simulink model "Copy_of_Facies"  (R2023a)
settings: Solver=VariableStepAuto  StartTime=0.0  StopTime=6  RelTol=1e-3
(part 1 of 2)
settings Model: Creator=Stefano  LastModifiedBy=stefanopanzieri
settings SolverCC: AlgebraicLoopSolver=TrustRegion
settings DebuggingCC: UnconnectedInputMsg=warning  UnconnectedOutputMsg=warning  UnconnectedLineMsg=warning
settings ModelReferenceCC: EnableRefExpFcnMdlSchedulingChecks=on
settings SFSimCC: CustomCodeUndefinedFunction=UseInterfaceOnly
settings RTWCC: DLArmComputeVersion=19.05

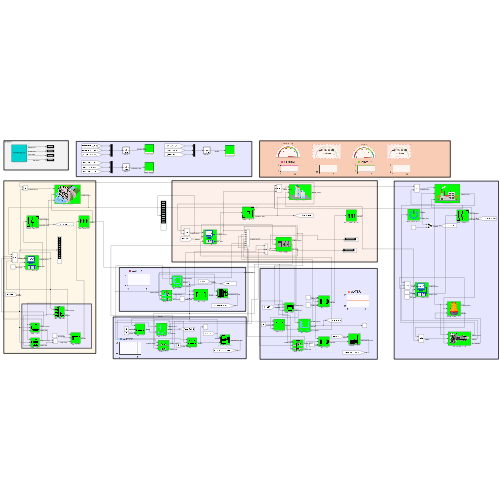
[thumbnail: Simulink's stored preview of the top-level diagram]
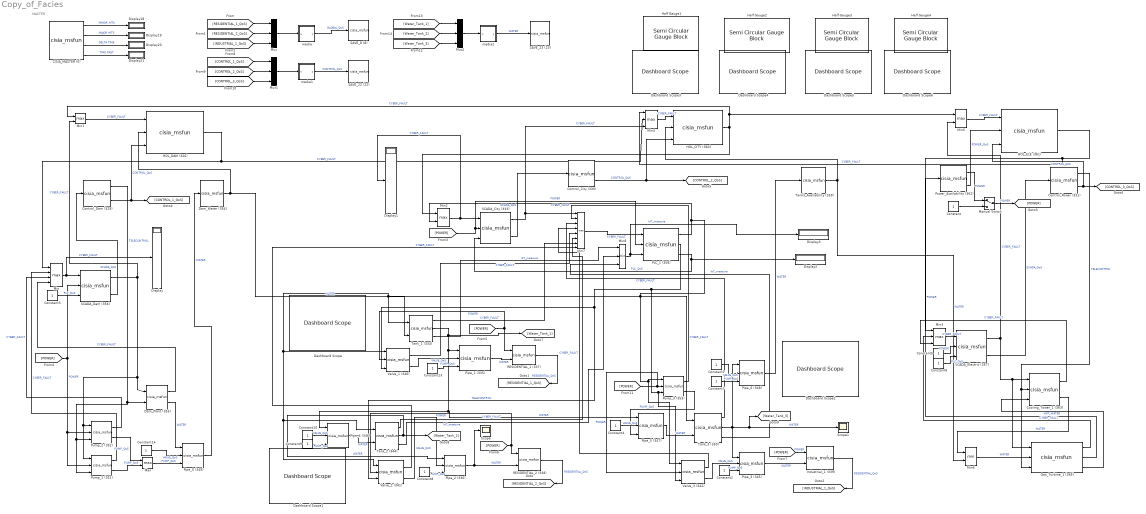
== system Copy_of_Facies ==
  note: MASTER
  CISIA_MASTER (0) : M-S-Function  FunctionName=cisia_msfun  Parameters=Parameter1, Parameter2, Parameter3, resources, Parameter4, Parameter5, Parameter6, Parameter7, Parameter8, Parameter9,Parameter11  mask(S-function:msfcn_unit_delay){Parameter1='CISIA_MASTER', Parameter2=1, Parameter3='SistemiIoT', resources=off, Parameter4=on, Parameter5=off, Parameter6=off, Parameter7=off, Parameter8=0.001, Parameter9=off, Parameter11=on}
      mask prompts: Parameter1 "entity name"; Parameter2 "sampling time"; Parameter3 "project"; resources "Save status at each major hit"; Parameter4 "Show Operative Levels with colors"; Parameter5 "Load Entities from file"; Parameter6 "Load Start from Mask"; Parameter7 "Real Time"; Parameter8 "Real Time Hit (sec)"; Parameter9 "Skip saving"; Parameter11 "Show unconnected"
      mask help: This is a level-2 MATLAB file S-function which demonstrates CISIA entity
      mask Display: disp('MASTER BLOCK')
  Constant{,1..10,13..14} (13 alike) : Constant
  Control_City (330) : M-S-Function  FunctionName=cisia_msfun  Parameters=Parameter1, Parameter2, Parameter3, resources, Parameter10, codeupdate, step_received, step_computed, dynamic_computed, step_sended, id_entity, id_project, id_type, name_type, color  mask(S-function:msfcn_unit_delay){Parameter1='Control_City', Parameter2=1, Parameter3='', resources=, Parameter10=off, codeupdate=off, step_received=|, step_computed=, dynamic_computed=, step_sended=|, id_entity=330, id_project=6, id_type=81, name_type=Control_Service, color=#FFFFFF}
      mask step_received=|
      | Control_Fault=1-SCADA_QoS;
      |
      | Operative_Level=1-Control_Fault;
      mask step_sended=|
      | TELECONTROL=1-Control_Fault;
      | CONTROL_QoS=1-Control_Fault;
      mask prompts: Parameter1 "entity name"; Parameter2 "sampling time"; Parameter3 "project"; resources "input resources and state variables"; Parameter10 "Bring state variables to output"; codeupdate "update code from mask"
      mask help: This is a level-2 MATLAB file S-function which demonstrates CISIA entity
      mask DialogControl Container1 Prompt: All parameters
      mask Display: image('Icons/Control_Service.png')
  Control_Dam (329) : M-S-Function  FunctionName=cisia_msfun  Parameters=Parameter1, Parameter2, Parameter3, resources, Parameter10, codeupdate, step_received, step_computed, dynamic_computed, step_sended, id_entity, id_project, id_type, name_type, color  mask(S-function:msfcn_unit_delay){Parameter1='Control_Dam', Parameter2=1, Parameter3='', resources=, Parameter10=off, codeupdate=off, step_received=|, step_computed=, dynamic_computed=, step_sended=|, id_entity=329, id_project=6, id_type=81, name_type=Control_Service, color=#FFFFFF}
      mask step_received=|
      | Control_Fault=1-SCADA_QoS;
      |
      | Operative_Level=1-Control_Fault;
      mask step_sended=|
      | TELECONTROL=1-Control_Fault;
      | CONTROL_QoS=1-Control_Fault;
      mask prompts: Parameter1 "entity name"; Parameter2 "sampling time"; Parameter3 "project"; resources "input resources and state variables"; Parameter10 "Bring state variables to output"; codeupdate "update code from mask"
      mask help: This is a level-2 MATLAB file S-function which demonstrates CISIA entity
      mask DialogControl Container1 Prompt: All parameters
      mask Display: image('Icons/Control_Service.png')
  Control_Power (331) : M-S-Function  FunctionName=cisia_msfun  Parameters=Parameter1, Parameter2, Parameter3, resources, Parameter10, codeupdate, step_received, step_computed, dynamic_computed, step_sended, id_entity, id_project, id_type, name_type, color  mask(S-function:msfcn_unit_delay){Parameter1='Control_Power', Parameter2=1, Parameter3='', resources=, Parameter10=off, codeupdate=off, step_received=|, step_computed=, dynamic_computed=, step_sended=|, id_entity=331, id_project=6, id_type=81, name_type=Control_Service, color=#FFFFFF}
      mask step_received=|
      | Control_Fault=1-SCADA_QoS;
      |
      | Operative_Level=1-Control_Fault;
      mask step_sended=|
      | TELECONTROL=1-Control_Fault;
      | CONTROL_QoS=1-Control_Fault;
      mask prompts: Parameter1 "entity name"; Parameter2 "sampling time"; Parameter3 "project"; resources "input resources and state variables"; Parameter10 "Bring state variables to output"; codeupdate "update code from mask"
      mask help: This is a level-2 MATLAB file S-function which demonstrates CISIA entity
      mask DialogControl Container1 Prompt: All parameters
      mask Display: image('Icons/Control_Service.png')
  Cooling_Tower_1 (363) : M-S-Function  FunctionName=cisia_msfun  Parameters=Parameter1, Parameter2, Parameter3, resources, Parameter10, codeupdate, step_received, step_computed, dynamic_computed, step_sended, id_entity, id_project, id_type, name_type, color  mask(S-function:msfcn_unit_delay){Parameter1='Cooling_Tower_1', Parameter2=1, Parameter3='', resources=, Parameter10=off, codeupdate=off, step_received=|, step_computed=, dynamic_computed=, step_sended=|, id_entity=363, id_project=6, id_type=92, name_type=CoolingTower, color=#FFFFFF}
      mask step_received=|
      | Cyber_Fault=max(CYBER_FAULT, transpose([Dos_attack MITM_attack Virus_Attack Port_Scan_Attack  BGP_hijacking BotNet_Attack Data_Corruption SW_Change Config_Change Port_Saturation]));
      |
      | Water_Fault=1-HOT_WATER;
      |
      | Operative_Level=min([1-max(Cyber_Fault) 1-Mechanical_Fault TELECONTROL]);
      mask step_sended=|
      | CYBER_FAULT=Cyber_Fault.*transpose([0 0 0.5 0.2 0 0 0 0 0 0]);
      |
      | WATER=Operative_Level;
      mask prompts: Parameter1 "entity name"; Parameter2 "sampling time"; Parameter3 "project"; resources "input resources and state variables"; Parameter10 "Bring state variables to output"; codeupdate "update code from mask"
      mask help: This is a level-2 MATLAB file S-function which demonstrates CISIA entity
      mask DialogControl Container1 Prompt: All parameters
      mask Display: image('Icons/CoolingTower.png')
  Dam_Plant (355) : M-S-Function  FunctionName=cisia_msfun  Parameters=Parameter1, Parameter2, Parameter3, resources, Parameter10, codeupdate, step_received, step_computed, dynamic_computed, step_sended, id_entity, id_project, id_type, name_type, color  mask(S-function:msfcn_unit_delay){Parameter1='Dam_Plant', Parameter2=1, Parameter3='', resources=, Parameter10=off, codeupdate=off, step_received=|, step_computed=, dynamic_computed=, step_sended=|, id_entity=355, id_project=6, id_type=88, name_type=Dam, color=#FFFFFF}
      mask step_received=|
      | Cyber_Fault=max(CYBER_FAULT, transpose([Dos_attack MITM_attack Virus_Attack Port_Scan_Attack  BGP_hijacking BotNet_Attack Data_Corruption SW_Change Config_Change Port_Saturation]));
      |
      |
      | Control_Fault=max([1-TELECONTROL Mechanical_Fault Dos_attack min(0.5,max(Cyber_Fault))]);
      |
      |
      |
      | Operative_Level=min([1-max(Cyber_Fault) 1-Mechanical_Fault 1-Control_Fault]);
      mask step_sended=|
      | CYBER_FAULT=Cyber_Fault.*transpose([0 0 0.5 0.2 0 0 0 0 0 0]);
      |
      | WATER=Operative_Level;
      mask prompts: Parameter1 "entity name"; Parameter2 "sampling time"; Parameter3 "project"; resources "input resources and state variables"; Parameter10 "Bring state variables to output"; codeupdate "update code from mask"
      mask help: This is a level-2 MATLAB file S-function which demonstrates CISIA entity
      mask DialogControl Container1 Prompt: All parameters
      mask Display: image('Icons/Dam.png')
  Dam_Water (354) : M-S-Function  FunctionName=cisia_msfun  Parameters=Parameter1, Parameter2, Parameter3, resources, Parameter10, codeupdate, step_received, step_computed, dynamic_computed, step_sended, id_entity, id_project, id_type, name_type, color  mask(S-function:msfcn_unit_delay){Parameter1='Dam_Water', Parameter2=1, Parameter3='', resources=, Parameter10=off, codeupdate=off, step_received=|, step_computed=, dynamic_computed=, step_sended=WATER=1-Water_Fault;, id_entity=354, id_project=6, id_type=95, name_type=Water_Availability, color=#FFFFFF}
      mask step_received=|
      | Water_Fault=1-WATER;
      |
      | Operative_Level=1-Water_Fault;
      mask prompts: Parameter1 "entity name"; Parameter2 "sampling time"; Parameter3 "project"; resources "input resources and state variables"; Parameter10 "Bring state variables to output"; codeupdate "update code from mask"
      mask help: This is a level-2 MATLAB file S-function which demonstrates CISIA entity
      mask DialogControl Container1 Prompt: All parameters
      mask Display: image('Icons/Water_Availability.png')
  Dashboard Scope{,1..6} (7 alike) : DashboardScope  Ymin=0  Ymax=1
  Display{,1..3,18..21} (8 alike) : Display
  Gas_Turbine_1 (365) : M-S-Function  FunctionName=cisia_msfun  Parameters=Parameter1, Parameter2, Parameter3, resources, Parameter10, codeupdate, step_received, step_computed, dynamic_computed, step_sended, id_entity, id_project, id_type, name_type, color  mask(S-function:msfcn_unit_delay){Parameter1='Gas_Turbine_1', Parameter2=1, Parameter3='', resources=, Parameter10=off, codeupdate=off, step_received=|, step_computed=, dynamic_computed=, step_sended=|, id_entity=365, id_project=6, id_type=99, name_type=Gas_Turbine, color=#FFFFFF}
      mask step_received=|
      | Cyber_Fault=max(CYBER_FAULT, transpose([Dos_attack MITM_attack Virus_Attack Port_Scan_Attack  BGP_hijacking BotNet_Attack Data_Corruption SW_Change Config_Change Port_Saturation]));
      |
      | Water_Fault=1-WATER;
      |
      | Operative_Level=min([1-max(Cyber_Fault) 1-Mechanical_Fault TELECONTROL 1-Water_Fault]);
      mask step_sended=|
      | CYBER_FAULT=Cyber_Fault.*transpose([0 0 0.5 0.2 0 0 0 0 0 0]);
      |
      | HOT_WATER=Operative_Level;
      |
      | POWER=Operative_Level;
      mask prompts: Parameter1 "entity name"; Parameter2 "sampling time"; Parameter3 "project"; resources "input resources and state variables"; Parameter10 "Bring state variables to output"; codeupdate "update code from mask"
      mask help: This is a level-2 MATLAB file S-function which demonstrates CISIA entity
      mask DialogControl Container1 Prompt: All parameters
      mask Display: image('Icons/Gas_Turbine.png')
  HOL_CITY (360) : M-S-Function  FunctionName=cisia_msfun  Parameters=Parameter1, Parameter2, Parameter3, resources, Parameter10, codeupdate, step_received, step_computed, dynamic_computed, step_sended, id_entity, id_project, id_type, name_type, color  mask(S-function:msfcn_unit_delay){Parameter1='HOL_CITY', Parameter2=1, Parameter3='', resources=, Parameter10=off, codeupdate=off, step_received=|, step_computed=, dynamic_computed=, step_sended=CYBER_FAULT=Cyber_Fault;, id_entity=360, id_project=6, id_type=96, name_type=HOL_CITY, color=#FFFFFF}
      mask step_received=|
      | Cyber_Fault=CYBER_FAULT;
      |
      | Operative_Level=min([1-max(CYBER_FAULT) WATER CONTROL_QoS]);
      mask prompts: Parameter1 "entity name"; Parameter2 "sampling time"; Parameter3 "project"; resources "input resources and state variables"; Parameter10 "Bring state variables to output"; codeupdate "update code from mask"
      mask help: This is a level-2 MATLAB file S-function which demonstrates CISIA entity
      mask DialogControl Container1 Prompt: All parameters
      mask Display: image('Icons/HOL_CITY.png')
  HOL_DAM (326) : M-S-Function  FunctionName=cisia_msfun  Parameters=Parameter1, Parameter2, Parameter3, resources, Parameter10, codeupdate, step_received, step_computed, dynamic_computed, step_sended, id_entity, id_project, id_type, name_type, color  mask(S-function:msfcn_unit_delay){Parameter1='HOL_DAM', Parameter2=1, Parameter3='', resources=, Parameter10=off, codeupdate=off, step_received=|, step_computed=, dynamic_computed=, step_sended=CYBER_FAULT=Cyber_Fault;, id_entity=326, id_project=6, id_type=78, name_type=HOL_DAM, color=#FFFFFF}
      mask step_received=|
      | Cyber_Fault=CYBER_FAULT;
      |
      | Operative_Level=min([1-max(CYBER_FAULT) WATER CONTROL_QoS]);
      mask prompts: Parameter1 "entity name"; Parameter2 "sampling time"; Parameter3 "project"; resources "input resources and state variables"; Parameter10 "Bring state variables to output"; codeupdate "update code from mask"
      mask help: This is a level-2 MATLAB file S-function which demonstrates CISIA entity
      mask DialogControl Container1 Prompt: All parameters
      mask Display: image('Icons/HOL_DAM.png')
  HOL_ELE (361) : M-S-Function  FunctionName=cisia_msfun  Parameters=Parameter1, Parameter2, Parameter3, resources, Parameter10, codeupdate, step_received, step_computed, dynamic_computed, step_sended, id_entity, id_project, id_type, name_type, color  mask(S-function:msfcn_unit_delay){Parameter1='HOL_ELE', Parameter2=1, Parameter3='', resources=, Parameter10=off, codeupdate=off, step_received=|, step_computed=, dynamic_computed=, step_sended=CYBER_FAULT=Cyber_Fault;, id_entity=361, id_project=6, id_type=97, name_type=HOL_ELE, color=#FFFFFF}
      mask step_received=|
      | Cyber_Fault=CYBER_FAULT;
      |
      | Operative_Level=min([1-max(CYBER_FAULT) POWER_QoS CONTROL_QoS]);
      mask prompts: Parameter1 "entity name"; Parameter2 "sampling time"; Parameter3 "project"; resources "input resources and state variables"; Parameter10 "Bring state variables to output"; codeupdate "update code from mask"
      mask help: This is a level-2 MATLAB file S-function which demonstrates CISIA entity
      mask DialogControl Container1 Prompt: All parameters
      mask Display: image('Icons/HOL_ELE.png')
  Half Gauge{1..4} (4 alike) : SemiCircularGaugeBlock  ScaleMax=1
  Industrial_1 (339) : M-S-Function  FunctionName=cisia_msfun  Parameters=Parameter1, Parameter2, Parameter3, resources, Parameter10, codeupdate, step_received, step_computed, dynamic_computed, step_sended, id_entity, id_project, id_type, name_type, color  mask(S-function:msfcn_unit_delay){Parameter1='Industrial_1', Parameter2=1, Parameter3='', resources=, Parameter10=off, codeupdate=off, step_received=|, step_computed=, dynamic_computed=, step_sended=RESIDENTIAL_QoS=Operative_Level;, id_entity=339, id_project=6, id_type=89, name_type=Residential, color=#FFFFFF}
      mask step_received=|
      | Power_Fault=1-POWER;
      | Water_Fault=1-WATER;
      |
      | Operative_Level=min(1-Power_Fault,1-Water_Fault);
      mask prompts: Parameter1 "entity name"; Parameter2 "sampling time"; Parameter3 "project"; resources "input resources and state variables"; Parameter10 "Bring state variables to output"; codeupdate "update code from mask"
      mask help: This is a level-2 MATLAB file S-function which demonstrates CISIA entity
      mask DialogControl Container1 Prompt: All parameters
      mask Display: image('Icons/Industrial_1.png')
  Manual Switch : ManualSwitch
  Max : MinMax  Function=max  Inputs=2
  Min : MinMax  Function=max  Inputs=4
  Min1 : MinMax  Function=max  Inputs=2
  Min2 : MinMax  Function=max  Inputs=2
  Min3 : MinMax  Function=max  Inputs=3
  Min4 : MinMax  Function=max  Inputs=3
  Min5 : MinMax  Function=max  Inputs=2
  Min6 : MinMax  Inputs=2
  Min7 : MinMax  Function=max  Inputs=8
  Min8 : MinMax  Inputs=3
  Mux : Mux  Inputs=3
  Mux1 : Mux  Inputs=3
  Mux2 : Mux  Inputs=3
  PLC_1 (358) : M-S-Function  FunctionName=cisia_msfun  Parameters=Parameter1, Parameter2, Parameter3, resources, Parameter10, codeupdate, step_received, step_computed, dynamic_computed, step_sended, id_entity, id_project, id_type, name_type, color  mask(S-function:msfcn_unit_delay){Parameter1='PLC_1', Parameter2=1, Parameter3='', resources=, Parameter10=off, codeupdate=off, step_received=|, step_computed=, dynamic_computed=, step_sended=|, id_entity=358, id_project=6, id_type=83, name_type=PLC, color=#FFFFFF}
      mask step_received=|
      | Cyber_Fault=max(CYBER_FAULT, transpose([Dos_attack MITM_attack Virus_Attack Port_Scan_Attack  BGP_hijacking BotNet_Attack Data_Corruption SW_Change Config_Change Port_Saturation]));
      |
      |
      | Control_Fault=max([1-IoT_measure Mechanical_Fault 1-POWER Dos_attack min(0.5,max(Cyber_Fault))]);
      |
      |
      |
      | Operative_Level=min([1-max(Cyber_Fault) 1-Mechanical_Fault 1-Control_Fault]);
      mask step_sended=|
      | CYBER_FAULT=Cyber_Fault.*transpose([0 0 0.5 0.2 0 0 0 0 0 0]);
      |
      | TELECONTROL=1-Control_Fault;
      | PLC_QoS=Operative_Level;
      mask prompts: Parameter1 "entity name"; Parameter2 "sampling time"; Parameter3 "project"; resources "input resources and state variables"; Parameter10 "Bring state variables to output"; codeupdate "update code from mask"
      mask help: This is a level-2 MATLAB file S-function which demonstrates CISIA entity
      mask DialogControl Container1 Prompt: All parameters
      mask Display: image('Icons/PLC.png')
  Pipe_0 (349) : M-S-Function  FunctionName=cisia_msfun  Parameters=Parameter1, Parameter2, Parameter3, resources, Parameter10, codeupdate, step_received, step_computed, dynamic_computed, step_sended, id_entity, id_project, id_type, name_type, color  mask(S-function:msfcn_unit_delay){Parameter1='Pipe_0', Parameter2=1, Parameter3='', resources=, Parameter10=off, codeupdate=off, step_received=|, step_computed=, dynamic_computed=, step_sended=WATER=1-Water_Fault;, id_entity=349, id_project=6, id_type=84, name_type=Pipe, color=#00FFFF}
      mask step_received=|
      | Water_Fault=max([1-WATER Mechanical_Fault 1-VALVE_QoS 1-PUMP_QoS]);
      |
      | Operative_Level=1-Mechanical_Fault;
      mask prompts: Parameter1 "entity name"; Parameter2 "sampling time"; Parameter3 "project"; resources "input resources and state variables"; Parameter10 "Bring state variables to output"; codeupdate "update code from mask"
      mask help: This is a level-2 MATLAB file S-function which demonstrates CISIA entity
      mask DialogControl Container1 Prompt: All parameters
      mask Display: image('Icons/Pipe.png')
  Pipe_1 (335) : M-S-Function  FunctionName=cisia_msfun  Parameters=Parameter1, Parameter2, Parameter3, resources, Parameter10, codeupdate, step_received, step_computed, dynamic_computed, step_sended, id_entity, id_project, id_type, name_type, color  mask(S-function:msfcn_unit_delay){Parameter1='Pipe_1', Parameter2=1, Parameter3='', resources=, Parameter10=off, codeupdate=off, step_received=|, step_computed=, dynamic_computed=, step_sended=WATER=1-Water_Fault;, id_entity=335, id_project=6, id_type=84, name_type=Pipe, color=#00FFFF}
      mask step_received=|
      | Water_Fault=max([1-WATER Mechanical_Fault 1-VALVE_QoS 1-PUMP_QoS]);
      |
      | Operative_Level=1-Mechanical_Fault;
      mask prompts: Parameter1 "entity name"; Parameter2 "sampling time"; Parameter3 "project"; resources "input resources and state variables"; Parameter10 "Bring state variables to output"; codeupdate "update code from mask"
      mask help: This is a level-2 MATLAB file S-function which demonstrates CISIA entity
      mask DialogControl Container1 Prompt: All parameters
      mask Display: image('Icons/Pipe.png')
  Pipe_2 (336) : M-S-Function  FunctionName=cisia_msfun  Parameters=Parameter1, Parameter2, Parameter3, resources, Parameter10, codeupdate, step_received, step_computed, dynamic_computed, step_sended, id_entity, id_project, id_type, name_type, color  mask(S-function:msfcn_unit_delay){Parameter1='Pipe_2', Parameter2=1, Parameter3='', resources=, Parameter10=off, codeupdate=off, step_received=|, step_computed=, dynamic_computed=, step_sended=WATER=1-Water_Fault;, id_entity=336, id_project=6, id_type=84, name_type=Pipe, color=#00FFFF}
      mask step_received=|
      | Water_Fault=max([1-WATER Mechanical_Fault 1-VALVE_QoS 1-PUMP_QoS]);
      |
      | Operative_Level=1-Mechanical_Fault;
      mask prompts: Parameter1 "entity name"; Parameter2 "sampling time"; Parameter3 "project"; resources "input resources and state variables"; Parameter10 "Bring state variables to output"; codeupdate "update code from mask"
      mask help: This is a level-2 MATLAB file S-function which demonstrates CISIA entity
      mask DialogControl Container1 Prompt: All parameters
      mask Display: image('Icons/Pipe.png')
  Pipe_3 (345) : M-S-Function  FunctionName=cisia_msfun  Parameters=Parameter1, Parameter2, Parameter3, resources, Parameter10, codeupdate, step_received, step_computed, dynamic_computed, step_sended, id_entity, id_project, id_type, name_type, color  mask(S-function:msfcn_unit_delay){Parameter1='Pipe_3', Parameter2=1, Parameter3='', resources=, Parameter10=off, codeupdate=off, step_received=|, step_computed=, dynamic_computed=, step_sended=WATER=1-Water_Fault;, id_entity=345, id_project=6, id_type=84, name_type=Pipe, color=#00FFFF}
      mask step_received=|
      | Water_Fault=max([1-WATER Mechanical_Fault 1-VALVE_QoS 1-PUMP_QoS]);
      |
      | Operative_Level=1-Mechanical_Fault;
      mask prompts: Parameter1 "entity name"; Parameter2 "sampling time"; Parameter3 "project"; resources "input resources and state variables"; Parameter10 "Bring state variables to output"; codeupdate "update code from mask"
      mask help: This is a level-2 MATLAB file S-function which demonstrates CISIA entity
      mask DialogControl Container1 Prompt: All parameters
      mask Display: image('Icons/Pipe.png')
  Pipe_4 (346) : M-S-Function  FunctionName=cisia_msfun  Parameters=Parameter1, Parameter2, Parameter3, resources, Parameter10, codeupdate, step_received, step_computed, dynamic_computed, step_sended, id_entity, id_project, id_type, name_type, color  mask(S-function:msfcn_unit_delay){Parameter1='Pipe_4', Parameter2=1, Parameter3='', resources=, Parameter10=off, codeupdate=off, step_received=|, step_computed=, dynamic_computed=, step_sended=WATER=1-Water_Fault;, id_entity=346, id_project=6, id_type=84, name_type=Pipe, color=#00FFFF}
      mask step_received=|
      | Water_Fault=max([1-WATER Mechanical_Fault 1-VALVE_QoS 1-PUMP_QoS]);
      |
      | Operative_Level=1-Mechanical_Fault;
      mask prompts: Parameter1 "entity name"; Parameter2 "sampling time"; Parameter3 "project"; resources "input resources and state variables"; Parameter10 "Bring state variables to output"; codeupdate "update code from mask"
      mask help: This is a level-2 MATLAB file S-function which demonstrates CISIA entity
      mask DialogControl Container1 Prompt: All parameters
      mask Display: image('Icons/Pipe.png')
  Pipe_5 (347) : M-S-Function  FunctionName=cisia_msfun  Parameters=Parameter1, Parameter2, Parameter3, resources, Parameter10, codeupdate, step_received, step_computed, dynamic_computed, step_sended, id_entity, id_project, id_type, name_type, color  mask(S-function:msfcn_unit_delay){Parameter1='Pipe_5', Parameter2=1, Parameter3='', resources=, Parameter10=off, codeupdate=off, step_received=|, step_computed=, dynamic_computed=, step_sended=WATER=1-Water_Fault;, id_entity=347, id_project=6, id_type=84, name_type=Pipe, color=#00FFFF}
      mask step_received=|
      | Water_Fault=max([1-WATER Mechanical_Fault 1-VALVE_QoS 1-PUMP_QoS]);
      |
      | Operative_Level=1-Mechanical_Fault;
      mask prompts: Parameter1 "entity name"; Parameter2 "sampling time"; Parameter3 "project"; resources "input resources and state variables"; Parameter10 "Bring state variables to output"; codeupdate "update code from mask"
      mask help: This is a level-2 MATLAB file S-function which demonstrates CISIA entity
      mask DialogControl Container1 Prompt: All parameters
      mask Display: image('Icons/Pipe.png')
  Pipe_6 (348) : M-S-Function  FunctionName=cisia_msfun  Parameters=Parameter1, Parameter2, Parameter3, resources, Parameter10, codeupdate, step_received, step_computed, dynamic_computed, step_sended, id_entity, id_project, id_type, name_type, color  mask(S-function:msfcn_unit_delay){Parameter1='Pipe_6', Parameter2=1, Parameter3='', resources=, Parameter10=off, codeupdate=off, step_received=|, step_computed=, dynamic_computed=, step_sended=WATER=1-Water_Fault;, id_entity=348, id_project=6, id_type=84, name_type=Pipe, color=#00FFFF}
      mask step_received=|
      | Water_Fault=max([1-WATER Mechanical_Fault 1-VALVE_QoS 1-PUMP_QoS]);
      |
      | Operative_Level=1-Mechanical_Fault;
      mask prompts: Parameter1 "entity name"; Parameter2 "sampling time"; Parameter3 "project"; resources "input resources and state variables"; Parameter10 "Bring state variables to output"; codeupdate "update code from mask"
      mask help: This is a level-2 MATLAB file S-function which demonstrates CISIA entity
      mask DialogControl Container1 Prompt: All parameters
      mask Display: image('Icons/Pipe.png')
  Power_Availability (362) : M-S-Function  FunctionName=cisia_msfun  Parameters=Parameter1, Parameter2, Parameter3, resources, Parameter10, codeupdate, step_received, step_computed, dynamic_computed, step_sended, id_entity, id_project, id_type, name_type, color  mask(S-function:msfcn_unit_delay){Parameter1='Power_Availability', Parameter2=1, Parameter3='', resources=, Parameter10=off, codeupdate=off, step_received=|, step_computed=, dynamic_computed=, step_sended=|, id_entity=362, id_project=6, id_type=94, name_type=PowerAvailability, color=#FFFFFF}
      mask step_received=|
      | Power_Fault=1-POWER;
      | Operative_Level=1-Power_Fault;
      mask step_sended=|
      | POWER=1-Power_Fault;
      | POWER_QoS=1-Power_Fault;
      mask prompts: Parameter1 "entity name"; Parameter2 "sampling time"; Parameter3 "project"; resources "input resources and state variables"; Parameter10 "Bring state variables to output"; codeupdate "update code from mask"
      mask help: This is a level-2 MATLAB file S-function which demonstrates CISIA entity
      mask DialogControl Container1 Prompt: All parameters
      mask Display: image('Icons/PowerAvailability.png')
  Pump_1 (351) : M-S-Function  FunctionName=cisia_msfun  Parameters=Parameter1, Parameter2, Parameter3, resources, Parameter10, codeupdate, step_received, step_computed, dynamic_computed, step_sended, id_entity, id_project, id_type, name_type, color  mask(S-function:msfcn_unit_delay){Parameter1='Pump_1', Parameter2=1, Parameter3='', resources=, Parameter10=off, codeupdate=off, step_received=|, step_computed=, dynamic_computed=, step_sended=|, id_entity=351, id_project=6, id_type=85, name_type=Pump, color=#FFFFFF}
      mask step_received=|
      | Cyber_Fault=max(CYBER_FAULT, transpose([Dos_attack MITM_attack Virus_Attack Port_Scan_Attack  BGP_hijacking BotNet_Attack Data_Corruption SW_Change Config_Change Port_Saturation]));
      |
      |
      | Control_Fault=max([1-TELECONTROL Mechanical_Fault Dos_attack min(0.5,max(Cyber_Fault))]);
      |
      |
      |
      | Operative_Level=min([1-max(Cyber_Fault) 1-Mechanical_Fault POWER]);
      mask step_sended=|
      | PUMP_QoS=1-Control_Fault;
      | CYBER_FAULT=Cyber_Fault.*transpose([0 0 0.5 0.2 0 0 0 0 0 0]);
      mask prompts: Parameter1 "entity name"; Parameter2 "sampling time"; Parameter3 "project"; resources "input resources and state variables"; Parameter10 "Bring state variables to output"; codeupdate "update code from mask"
      mask help: This is a level-2 MATLAB file S-function which demonstrates CISIA entity
      mask DialogControl Container1 Prompt: All parameters
      mask Display: image('Icons/Pump.png')
  Pump_2 (352) : M-S-Function  FunctionName=cisia_msfun  Parameters=Parameter1, Parameter2, Parameter3, resources, Parameter10, codeupdate, step_received, step_computed, dynamic_computed, step_sended, id_entity, id_project, id_type, name_type, color  mask(S-function:msfcn_unit_delay){Parameter1='Pump_2', Parameter2=1, Parameter3='', resources=, Parameter10=off, codeupdate=off, step_received=|, step_computed=, dynamic_computed=, step_sended=|, id_entity=352, id_project=6, id_type=85, name_type=Pump, color=#FFFFFF}
      mask step_received=|
      | Cyber_Fault=max(CYBER_FAULT, transpose([Dos_attack MITM_attack Virus_Attack Port_Scan_Attack  BGP_hijacking BotNet_Attack Data_Corruption SW_Change Config_Change Port_Saturation]));
      |
      |
      | Control_Fault=max([1-TELECONTROL Mechanical_Fault Dos_attack min(0.5,max(Cyber_Fault))]);
      |
      |
      |
      | Operative_Level=min([1-max(Cyber_Fault) 1-Mechanical_Fault POWER]);
      mask step_sended=|
      | PUMP_QoS=1-Control_Fault;
      | CYBER_FAULT=Cyber_Fault.*transpose([0 0 0.5 0.2 0 0 0 0 0 0]);
      mask prompts: Parameter1 "entity name"; Parameter2 "sampling time"; Parameter3 "project"; resources "input resources and state variables"; Parameter10 "Bring state variables to output"; codeupdate "update code from mask"
      mask help: This is a level-2 MATLAB file S-function which demonstrates CISIA entity
      mask DialogControl Container1 Prompt: All parameters
      mask Display: image('Icons/Pump.png')
  Pump_3 (353) : M-S-Function  FunctionName=cisia_msfun  Parameters=Parameter1, Parameter2, Parameter3, resources, Parameter10, codeupdate, step_received, step_computed, dynamic_computed, step_sended, id_entity, id_project, id_type, name_type, color  mask(S-function:msfcn_unit_delay){Parameter1='Pump_3', Parameter2=1, Parameter3='', resources=, Parameter10=off, codeupdate=off, step_received=|, step_computed=, dynamic_computed=, step_sended=|, id_entity=353, id_project=6, id_type=85, name_type=Pump, color=#FFFFFF}
      mask step_received=|
      | Cyber_Fault=max(CYBER_FAULT, transpose([Dos_attack MITM_attack Virus_Attack Port_Scan_Attack  BGP_hijacking BotNet_Attack Data_Corruption SW_Change Config_Change Port_Saturation]));
      |
      |
      | Control_Fault=max([1-TELECONTROL Mechanical_Fault Dos_attack min(0.5,max(Cyber_Fault))]);
      |
      |
      |
      | Operative_Level=min([1-max(Cyber_Fault) 1-Mechanical_Fault POWER]);
      mask step_sended=|
      | PUMP_QoS=1-Control_Fault;
      | CYBER_FAULT=Cyber_Fault.*transpose([0 0 0.5 0.2 0 0 0 0 0 0]);
      mask prompts: Parameter1 "entity name"; Parameter2 "sampling time"; Parameter3 "project"; resources "input resources and state variables"; Parameter10 "Bring state variables to output"; codeupdate "update code from mask"
      mask help: This is a level-2 MATLAB file S-function which demonstrates CISIA entity
      mask DialogControl Container1 Prompt: All parameters
      mask Display: image('Icons/Pump.png')
  RESIDENTIAL_1 (337) : M-S-Function  FunctionName=cisia_msfun  Parameters=Parameter1, Parameter2, Parameter3, resources, Parameter10, codeupdate, step_received, step_computed, dynamic_computed, step_sended, id_entity, id_project, id_type, name_type, color  mask(S-function:msfcn_unit_delay){Parameter1='RESIDENTIAL_1', Parameter2=1, Parameter3='', resources=, Parameter10=off, codeupdate=off, step_received=|, step_computed=, dynamic_computed=, step_sended=RESIDENTIAL_QoS=Operative_Level;, id_entity=337, id_project=6, id_type=89, name_type=Residential, color=#FFFFFF}
      mask step_received=|
      | Power_Fault=1-POWER;
      | Water_Fault=1-WATER;
      |
      | Operative_Level=min(1-Power_Fault,1-Water_Fault);
      mask prompts: Parameter1 "entity name"; Parameter2 "sampling time"; Parameter3 "project"; resources "input resources and state variables"; Parameter10 "Bring state variables to output"; codeupdate "update code from mask"
      mask help: This is a level-2 MATLAB file S-function which demonstrates CISIA entity
      mask DialogControl Container1 Prompt: All parameters
      mask Display: image('Icons/Residential.png')
  RESIDENTIAL_2 (338) : M-S-Function  FunctionName=cisia_msfun  Parameters=Parameter1, Parameter2, Parameter3, resources, Parameter10, codeupdate, step_received, step_computed, dynamic_computed, step_sended, id_entity, id_project, id_type, name_type, color  mask(S-function:msfcn_unit_delay){Parameter1='RESIDENTIAL_2', Parameter2=1, Parameter3='', resources=, Parameter10=off, codeupdate=off, step_received=|, step_computed=, dynamic_computed=, step_sended=RESIDENTIAL_QoS=Operative_Level;, id_entity=338, id_project=6, id_type=89, name_type=Residential, color=#FFFFFF}
      mask step_received=|
      | Power_Fault=1-POWER;
      | Water_Fault=1-WATER;
      |
      | Operative_Level=min(1-Power_Fault,1-Water_Fault);
      mask prompts: Parameter1 "entity name"; Parameter2 "sampling time"; Parameter3 "project"; resources "input resources and state variables"; Parameter10 "Bring state variables to output"; codeupdate "update code from mask"
      mask help: This is a level-2 MATLAB file S-function which demonstrates CISIA entity
      mask DialogControl Container1 Prompt: All parameters
      mask Display: image('Icons/Residential.png')
  SAVE_22 (22) : M-S-Function  FunctionName=cisia_msfun  Parameters=Parameter1, Parameter2, Parameter3, Parameter4,Parameter5,Parameter6,Parameter7  mask(S-function:msfcn_unit_delay){Parameter1='SAVE_22', Parameter2=1, Parameter3='SistemiIoT', Parameter4=on, Parameter5=[1], Parameter6=[1], Parameter7=off}
      mask prompts: Parameter1 "entity name"; Parameter2 "sampling time"; Parameter3 "project"; Parameter4 "display bars"; Parameter5 "values"; Parameter6 "logic"; Parameter7 "display B/W"
      mask help: This is a level-2 MATLAB file S-function which demonstrates CISIA entity
      mask DialogControl Container3 Prompt: Display
      mask Display:
      | display=get_param(gcb, 'Parameter4');
      | greymap=get_param(gcb, 'Parameter7');
      | 
      | if strcmp(display,'on')
      | 
      |     val=str2num(get_param(gcb, 'Parameter5'));
      |     logic=str2num(get_param(gcb, 'Parameter6'));
      |     n=length(val);
      | 
      |     val2=val;
      |     l=length(logic);
      |     if l>0
      |         for i=1:l
      |             if logic(i)==-1
      |                 val2(i)=1-val2(i);
      |             end
      |         end
      |     end
      | 
      | 
      | 
      | 
      |     if strcmp(greymap,'on')
      |         val_r=round(val2*50)+1;
      |         colormap=gray(60);
      |         color2=[0 0 0];
      |     else
      |         val_r=round(val2*20)+1;
      |         colormap=hsv(60);
      |         color2=[0 0 1];
      |     end
      | 
      |     patch([0 0 n n], [0 -0.2 -0.2 0], [1 1 1]);
      | 
      |     for i=1:n
      |         color=colormap(val_r(i),:);
      |         patch([i-1 i-1 i i],[0 1 1 0],color)
      |         patch([i-1 i],[val(i) val(i)],color2)
      | 
      |     end
      | 
      |     for i=1:n
      |         patch([i i], [-0.2 1], [0 0 0]);
      |         text(i-0.5, -0.1, num2str(val(i)));
      |     end
      | 
      | 
      | else
      | 
      |     disp('SAVE');
      | 
      | end
  SAVE_23 (23) : M-S-Function  FunctionName=cisia_msfun  Parameters=Parameter1, Parameter2, Parameter3, Parameter4,Parameter5,Parameter6,Parameter7  mask(S-function:msfcn_unit_delay){Parameter1='SAVE_23', Parameter2=1, Parameter3='SistemiIoT', Parameter4=on, Parameter5=[1], Parameter6=[1], Parameter7=off}
      mask prompts: Parameter1 "entity name"; Parameter2 "sampling time"; Parameter3 "project"; Parameter4 "display bars"; Parameter5 "values"; Parameter6 "logic"; Parameter7 "display B/W"
      mask help: This is a level-2 MATLAB file S-function which demonstrates CISIA entity
      mask DialogControl Container3 Prompt: Display
      mask Display:
      | display=get_param(gcb, 'Parameter4');
      | greymap=get_param(gcb, 'Parameter7');
      | 
      | if strcmp(display,'on')
      | 
      |     val=str2num(get_param(gcb, 'Parameter5'));
      |     logic=str2num(get_param(gcb, 'Parameter6'));
      |     n=length(val);
      | 
      |     val2=val;
      |     l=length(logic);
      |     if l>0
      |         for i=1:l
      |             if logic(i)==-1
      |                 val2(i)=1-val2(i);
      |             end
      |         end
      |     end
      | 
      | 
      | 
      | 
      |     if strcmp(greymap,'on')
      |         val_r=round(val2*50)+1;
      |         colormap=gray(60);
      |         color2=[0 0 0];
      |     else
      |         val_r=round(val2*20)+1;
      |         colormap=hsv(60);
      |         color2=[0 0 1];
      |     end
      | 
      |     patch([0 0 n n], [0 -0.2 -0.2 0], [1 1 1]);
      | 
      |     for i=1:n
      |         color=colormap(val_r(i),:);
      |         patch([i-1 i-1 i i],[0 1 1 0],color)
      |         patch([i-1 i],[val(i) val(i)],color2)
      | 
      |     end
      | 
      |     for i=1:n
      |         patch([i i], [-0.2 1], [0 0 0]);
      |         text(i-0.5, -0.1, num2str(val(i)));
      |     end
      | 
      | 
      | else
      | 
      |     disp('SAVE');
      | 
      | end
  SAVE_8 (8) : M-S-Function  FunctionName=cisia_msfun  Parameters=Parameter1, Parameter2, Parameter3, Parameter4,Parameter5,Parameter6,Parameter7  mask(S-function:msfcn_unit_delay){Parameter1='SAVE_8', Parameter2=1, Parameter3='SistemiIoT', Parameter4=on, Parameter5=[1], Parameter6=[1], Parameter7=off}
      mask prompts: Parameter1 "entity name"; Parameter2 "sampling time"; Parameter3 "project"; Parameter4 "display bars"; Parameter5 "values"; Parameter6 "logic"; Parameter7 "display B/W"
      mask help: This is a level-2 MATLAB file S-function which demonstrates CISIA entity
      mask DialogControl Container3 Prompt: Display
      mask Display:
      | display=get_param(gcb, 'Parameter4');
      | greymap=get_param(gcb, 'Parameter7');
      | 
      | if strcmp(display,'on')
      | 
      |     val=str2num(get_param(gcb, 'Parameter5'));
      |     logic=str2num(get_param(gcb, 'Parameter6'));
      |     n=length(val);
      | 
      |     val2=val;
      |     l=length(logic);
      |     if l>0
      |         for i=1:l
      |             if logic(i)==-1
      |                 val2(i)=1-val2(i);
      |             end
      |         end
      |     end
      | 
      | 
      | 
      | 
      |     if strcmp(greymap,'on')
      |         val_r=round(val2*50)+1;
      |         colormap=gray(60);
      |         color2=[0 0 0];
      |     else
      |         val_r=round(val2*20)+1;
      |         colormap=hsv(60);
      |         color2=[0 0 1];
      |     end
      | 
      |     patch([0 0 n n], [0 -0.2 -0.2 0], [1 1 1]);
      | 
      |     for i=1:n
      |         color=colormap(val_r(i),:);
      |         patch([i-1 i-1 i i],[0 1 1 0],color)
      |         patch([i-1 i],[val(i) val(i)],color2)
      | 
      |     end
      | 
      |     for i=1:n
      |         patch([i i], [-0.2 1], [0 0 0]);
      |         text(i-0.5, -0.1, num2str(val(i)));
      |     end
      | 
      | 
      | else
      | 
      |     disp('SAVE');
      | 
      | end
  SCADA_City (333) : M-S-Function  FunctionName=cisia_msfun  Parameters=Parameter1, Parameter2, Parameter3, resources, Parameter10, codeupdate, step_received, step_computed, dynamic_computed, step_sended, id_entity, id_project, id_type, name_type, color  mask(S-function:msfcn_unit_delay){Parameter1='SCADA_City', Parameter2=1, Parameter3='', resources=, Parameter10=off, codeupdate=off, step_received=|, step_computed=, dynamic_computed=, step_sended=|, id_entity=333, id_project=6, id_type=82, name_type=SCADA, color=#FFFFFF}
      mask step_received=|
      | Cyber_Fault=max(CYBER_FAULT, transpose([Dos_attack MITM_attack Virus_Attack Port_Scan_Attack  BGP_hijacking BotNet_Attack Data_Corruption SW_Change Config_Change Port_Saturation]));
      |
      |
      | Control_Fault=max([Mechanical_Fault Dos_attack min(0.5,max(Cyber_Fault))]);
      |
      |
      |
      | Operative_Level=min([1-max(Cyber_Fault) 1-Mechanical_Fault POWER PLC_QoS]);
      mask step_sended=|
      | SCADA_QoS=Operative_Level;
      |
      | CYBER_FAULT=Cyber_Fault.*transpose([0 0 0.5 0.2 0 0 0 0 0 0]);
      mask prompts: Parameter1 "entity name"; Parameter2 "sampling time"; Parameter3 "project"; resources "input resources and state variables"; Parameter10 "Bring state variables to output"; codeupdate "update code from mask"
      mask help: This is a level-2 MATLAB file S-function which demonstrates CISIA entity
      mask DialogControl Container1 Prompt: All parameters
      mask Display: image('Icons/SCADA.png')
  SCADA_Dam (356) : M-S-Function  FunctionName=cisia_msfun  Parameters=Parameter1, Parameter2, Parameter3, resources, Parameter10, codeupdate, step_received, step_computed, dynamic_computed, step_sended, id_entity, id_project, id_type, name_type, color  mask(S-function:msfcn_unit_delay){Parameter1='SCADA_Dam', Parameter2=1, Parameter3='', resources=, Parameter10=off, codeupdate=off, step_received=|, step_computed=, dynamic_computed=, step_sended=|, id_entity=356, id_project=6, id_type=82, name_type=SCADA, color=#FFFFFF}
      mask step_received=|
      | Cyber_Fault=max(CYBER_FAULT, transpose([Dos_attack MITM_attack Virus_Attack Port_Scan_Attack  BGP_hijacking BotNet_Attack Data_Corruption SW_Change Config_Change Port_Saturation]));
      |
      |
      | Control_Fault=max([Mechanical_Fault Dos_attack min(0.5,max(Cyber_Fault))]);
      |
      |
      |
      | Operative_Level=min([1-max(Cyber_Fault) 1-Mechanical_Fault POWER PLC_QoS]);
      mask step_sended=|
      | SCADA_QoS=Operative_Level;
      |
      | CYBER_FAULT=Cyber_Fault.*transpose([0 0 0.5 0.2 0 0 0 0 0 0]);
      mask prompts: Parameter1 "entity name"; Parameter2 "sampling time"; Parameter3 "project"; resources "input resources and state variables"; Parameter10 "Bring state variables to output"; codeupdate "update code from mask"
      mask help: This is a level-2 MATLAB file S-function which demonstrates CISIA entity
      mask DialogControl Container1 Prompt: All parameters
      mask Display: image('Icons/SCADA.png')
  SCADA_Electric (357) : M-S-Function  FunctionName=cisia_msfun  Parameters=Parameter1, Parameter2, Parameter3, resources, Parameter10, codeupdate, step_received, step_computed, dynamic_computed, step_sended, id_entity, id_project, id_type, name_type, color  mask(S-function:msfcn_unit_delay){Parameter1='SCADA_Electric', Parameter2=1, Parameter3='', resources=, Parameter10=off, codeupdate=off, step_received=|, step_computed=, dynamic_computed=, step_sended=|, id_entity=357, id_project=6, id_type=82, name_type=SCADA, color=#FFFFFF}
      mask step_received=|
      | Cyber_Fault=max(CYBER_FAULT, transpose([Dos_attack MITM_attack Virus_Attack Port_Scan_Attack  BGP_hijacking BotNet_Attack Data_Corruption SW_Change Config_Change Port_Saturation]));
      |
      |
      | Control_Fault=max([Mechanical_Fault Dos_attack min(0.5,max(Cyber_Fault))]);
      |
      |
      |
      | Operative_Level=min([1-max(Cyber_Fault) 1-Mechanical_Fault POWER PLC_QoS]);
      mask step_sended=|
      | SCADA_QoS=Operative_Level;
      |
      | CYBER_FAULT=Cyber_Fault.*transpose([0 0 0.5 0.2 0 0 0 0 0 0]);
      mask prompts: Parameter1 "entity name"; Parameter2 "sampling time"; Parameter3 "project"; resources "input resources and state variables"; Parameter10 "Bring state variables to output"; codeupdate "update code from mask"
      mask help: This is a level-2 MATLAB file S-function which demonstrates CISIA entity
      mask DialogControl Container1 Prompt: All parameters
      mask Display: image('Icons/SCADA.png')
  Scope : Scope
  Scope1 : Scope
  Tank3_Availability (359) : M-S-Function  FunctionName=cisia_msfun  Parameters=Parameter1, Parameter2, Parameter3, resources, Parameter10, codeupdate, step_received, step_computed, dynamic_computed, step_sended, id_entity, id_project, id_type, name_type, color  mask(S-function:msfcn_unit_delay){Parameter1='Tank3_Availability', Parameter2=1, Parameter3='', resources=, Parameter10=off, codeupdate=off, step_received=|, step_computed=, dynamic_computed=, step_sended=WATER=1-Water_Fault;, id_entity=359, id_project=6, id_type=95, name_type=Water_Availability, color=#FFFFFF}
      mask step_received=|
      | Water_Fault=1-WATER;
      |
      | Operative_Level=1-Water_Fault;
      mask prompts: Parameter1 "entity name"; Parameter2 "sampling time"; Parameter3 "project"; resources "input resources and state variables"; Parameter10 "Bring state variables to output"; codeupdate "update code from mask"
      mask help: This is a level-2 MATLAB file S-function which demonstrates CISIA entity
      mask DialogControl Container1 Prompt: All parameters
      mask Display: image('Icons/Water_Availability.png')
  Tank_1 (334) : M-S-Function  FunctionName=cisia_msfun  Parameters=Parameter1, Parameter2, Parameter3, resources, Parameter10, codeupdate, step_received, step_computed, dynamic_computed, step_sended, id_entity, id_project, id_type, name_type, color  mask(S-function:msfcn_unit_delay){Parameter1='Tank_1', Parameter2=1, Parameter3='', resources=, Parameter10=off, codeupdate=off, step_received=|, step_computed=Water_Level_new=max(0,Water_Level-0.2*Water_Fault);, dynamic_computed=, step_sended=|, id_entity=334, id_project=6, id_type=87, name_type=Tank, color=#FFFFFF}
      mask step_received=|
      | Cyber_Fault=max(CYBER_FAULT, transpose([Dos_attack MITM_attack Virus_Attack Port_Scan_Attack  BGP_hijacking BotNet_Attack Data_Corruption SW_Change Config_Change Port_Saturation]));
      |
      | Water_Fault=1-WATER;
      |
      | Operative_Level=min([1-max(Cyber_Fault) 1-Mechanical_Fault 1-IoT_Fault]);
      mask step_sended=|
      | WATER=Water_Level*Operative_Level;
      |
      | CYBER_FAULT=Cyber_Fault.*transpose([0 0 0.5 0.2 0 0 0 0 0 0]);
      |
      | IoT_measure=min([1-IoT_Fault  1-max(Cyber_Fault)]);
      mask prompts: Parameter1 "entity name"; Parameter2 "sampling time"; Parameter3 "project"; resources "input resources and state variables"; Parameter10 "Bring state variables to output"; codeupdate "update code from mask"
      mask help: This is a level-2 MATLAB file S-function which demonstrates CISIA entity
      mask DialogControl Container1 Prompt: All parameters
      mask Display: image('Icons/Tank.png')
  Tank_2 (344) : M-S-Function  FunctionName=cisia_msfun  Parameters=Parameter1, Parameter2, Parameter3, resources, Parameter10, codeupdate, step_received, step_computed, dynamic_computed, step_sended, id_entity, id_project, id_type, name_type, color  mask(S-function:msfcn_unit_delay){Parameter1='Tank_2', Parameter2=1, Parameter3='', resources=, Parameter10=off, codeupdate=off, step_received=|, step_computed=Water_Level_new=max(0,Water_Level-0.2*Water_Fault);, dynamic_computed=, step_sended=|, id_entity=344, id_project=6, id_type=87, name_type=Tank, color=#FFFFFF}
      mask step_received=|
      | Cyber_Fault=max(CYBER_FAULT, transpose([Dos_attack MITM_attack Virus_Attack Port_Scan_Attack  BGP_hijacking BotNet_Attack Data_Corruption SW_Change Config_Change Port_Saturation]));
      |
      | Water_Fault=1-WATER;
      |
      | Operative_Level=min([1-max(Cyber_Fault) 1-Mechanical_Fault 1-IoT_Fault]);
      mask step_sended=|
      | WATER=Water_Level*Operative_Level;
      |
      | CYBER_FAULT=Cyber_Fault.*transpose([0 0 0.5 0.2 0 0 0 0 0 0]);
      |
      | IoT_measure=min([1-IoT_Fault  1-max(Cyber_Fault)]);
      mask prompts: Parameter1 "entity name"; Parameter2 "sampling time"; Parameter3 "project"; resources "input resources and state variables"; Parameter10 "Bring state variables to output"; codeupdate "update code from mask"
      mask help: This is a level-2 MATLAB file S-function which demonstrates CISIA entity
      mask DialogControl Container1 Prompt: All parameters
      mask Display: image('Icons/Tank.png')
  Tank_3 (350) : M-S-Function  FunctionName=cisia_msfun  Parameters=Parameter1, Parameter2, Parameter3, resources, Parameter10, codeupdate, step_received, step_computed, dynamic_computed, step_sended, id_entity, id_project, id_type, name_type, color  mask(S-function:msfcn_unit_delay){Parameter1='Tank_3', Parameter2=1, Parameter3='', resources=, Parameter10=off, codeupdate=off, step_received=|, step_computed=Water_Level_new=max(0,Water_Level-0.2*Water_Fault);, dynamic_computed=, step_sended=|, id_entity=350, id_project=6, id_type=87, name_type=Tank, color=#FFFFFF}
      mask step_received=|
      | Cyber_Fault=max(CYBER_FAULT, transpose([Dos_attack MITM_attack Virus_Attack Port_Scan_Attack  BGP_hijacking BotNet_Attack Data_Corruption SW_Change Config_Change Port_Saturation]));
      |
      | Water_Fault=1-WATER;
      |
      | Operative_Level=min([1-max(Cyber_Fault) 1-Mechanical_Fault 1-IoT_Fault]);
      mask step_sended=|
      | WATER=Water_Level*Operative_Level;
      |
      | CYBER_FAULT=Cyber_Fault.*transpose([0 0 0.5 0.2 0 0 0 0 0 0]);
      |
      | IoT_measure=min([1-IoT_Fault  1-max(Cyber_Fault)]);
      mask prompts: Parameter1 "entity name"; Parameter2 "sampling time"; Parameter3 "project"; resources "input resources and state variables"; Parameter10 "Bring state variables to output"; codeupdate "update code from mask"
      mask help: This is a level-2 MATLAB file S-function which demonstrates CISIA entity
      mask DialogControl Container1 Prompt: All parameters
      mask Display: image('Icons/Tank.png')
  Valve_1 (340) : M-S-Function  FunctionName=cisia_msfun  Parameters=Parameter1, Parameter2, Parameter3, resources, Parameter10, codeupdate, step_received, step_computed, dynamic_computed, step_sended, id_entity, id_project, id_type, name_type, color  mask(S-function:msfcn_unit_delay){Parameter1='Valve_1', Parameter2=1, Parameter3='', resources=, Parameter10=off, codeupdate=off, step_received=|, step_computed=, dynamic_computed=, step_sended=|, id_entity=340, id_project=6, id_type=86, name_type=Valve, color=#FFFFFF}
      mask step_received=|
      | Cyber_Fault=max(CYBER_FAULT, transpose([Dos_attack MITM_attack Virus_Attack Port_Scan_Attack  BGP_hijacking BotNet_Attack Data_Corruption SW_Change Config_Change Port_Saturation]));
      |
      |
      | Control_Fault=max([1-TELECONTROL Mechanical_Fault Dos_attack min(0.5,max(Cyber_Fault))]);
      |
      |
      |
      | Operative_Level=min([1-max(Cyber_Fault) 1-Mechanical_Fault POWER]);
      mask step_sended=|
      | VALVE_QoS=Operative_Level;
      |
      | CYBER_FAULT=Cyber_Fault.*transpose([0 0 0.5 0.2 0 0 0 0 0 0]);
      mask prompts: Parameter1 "entity name"; Parameter2 "sampling time"; Parameter3 "project"; resources "input resources and state variables"; Parameter10 "Bring state variables to output"; codeupdate "update code from mask"
      mask help: This is a level-2 MATLAB file S-function which demonstrates CISIA entity
      mask DialogControl Container1 Prompt: All parameters
      mask Display: image('Icons/Valve.png')
  Valve_2 (341) : M-S-Function  FunctionName=cisia_msfun  Parameters=Parameter1, Parameter2, Parameter3, resources, Parameter10, codeupdate, step_received, step_computed, dynamic_computed, step_sended, id_entity, id_project, id_type, name_type, color  mask(S-function:msfcn_unit_delay){Parameter1='Valve_2', Parameter2=1, Parameter3='', resources=, Parameter10=off, codeupdate=off, step_received=|, step_computed=, dynamic_computed=, step_sended=|, id_entity=341, id_project=6, id_type=86, name_type=Valve, color=#FFFFFF}
      mask step_received=|
      | Cyber_Fault=max(CYBER_FAULT, transpose([Dos_attack MITM_attack Virus_Attack Port_Scan_Attack  BGP_hijacking BotNet_Attack Data_Corruption SW_Change Config_Change Port_Saturation]));
      |
      |
      | Control_Fault=max([1-TELECONTROL Mechanical_Fault Dos_attack min(0.5,max(Cyber_Fault))]);
      |
      |
      |
      | Operative_Level=min([1-max(Cyber_Fault) 1-Mechanical_Fault POWER]);
      mask step_sended=|
      | VALVE_QoS=Operative_Level;
      |
      | CYBER_FAULT=Cyber_Fault.*transpose([0 0 0.5 0.2 0 0 0 0 0 0]);
      mask prompts: Parameter1 "entity name"; Parameter2 "sampling time"; Parameter3 "project"; resources "input resources and state variables"; Parameter10 "Bring state variables to output"; codeupdate "update code from mask"
      mask help: This is a level-2 MATLAB file S-function which demonstrates CISIA entity
      mask DialogControl Container1 Prompt: All parameters
      mask Display: image('Icons/Valve.png')
  Valve_3 (342) : M-S-Function  FunctionName=cisia_msfun  Parameters=Parameter1, Parameter2, Parameter3, resources, Parameter10, codeupdate, step_received, step_computed, dynamic_computed, step_sended, id_entity, id_project, id_type, name_type, color  mask(S-function:msfcn_unit_delay){Parameter1='Valve_3', Parameter2=1, Parameter3='', resources=, Parameter10=off, codeupdate=off, step_received=|, step_computed=, dynamic_computed=, step_sended=|, id_entity=342, id_project=6, id_type=86, name_type=Valve, color=#FFFFFF}
      mask step_received=|
      | Cyber_Fault=max(CYBER_FAULT, transpose([Dos_attack MITM_attack Virus_Attack Port_Scan_Attack  BGP_hijacking BotNet_Attack Data_Corruption SW_Change Config_Change Port_Saturation]));
      |
      |
      | Control_Fault=max([1-TELECONTROL Mechanical_Fault Dos_attack min(0.5,max(Cyber_Fault))]);
      |
      |
      |
      | Operative_Level=min([1-max(Cyber_Fault) 1-Mechanical_Fault POWER]);
      mask step_sended=|
      | VALVE_QoS=Operative_Level;
      |
      | CYBER_FAULT=Cyber_Fault.*transpose([0 0 0.5 0.2 0 0 0 0 0 0]);
      mask prompts: Parameter1 "entity name"; Parameter2 "sampling time"; Parameter3 "project"; resources "input resources and state variables"; Parameter10 "Bring state variables to output"; codeupdate "update code from mask"
      mask help: This is a level-2 MATLAB file S-function which demonstrates CISIA entity
      mask DialogControl Container1 Prompt: All parameters
      mask Display: image('Icons/Valve.png')
  media : MATLAB Function  TreatAsAtomicUnit=on
  media1 : MATLAB Function  TreatAsAtomicUnit=on
  media2 : MATLAB Function  TreatAsAtomicUnit=on
  wires:
  media/1(y) -> SAVE_8 (8)/1  "GLOBAL_QoS"
  CISIA_MASTER (0)/1 -> Display18/1  "MINOR HITS"
  CISIA_MASTER (0)/2 -> Display19/1  "MAJOR HITS"
  CISIA_MASTER (0)/4 -> Display21/1  "TIME PAST"
  CISIA_MASTER (0)/3 -> Display20/1  "DELTA TIME"
  Pipe_2 (336)/1 -> Scope/1, RESIDENTIAL_2 (338)/2  "WATER"
  Mux/1 -> media/1(u)
  RESIDENTIAL_2 (338)/1 -> [RESIDENTIAL_2_QoS]  "RESIDENTIAL_QoS"
  [RESIDENTIAL_1_QoS] -> Mux/1
  [POWER] -> RESIDENTIAL_2 (338)/1, Valve_2 (341)/2  "POWER"
  Pipe_1 (335)/1 -> RESIDENTIAL_1 (337)/2  "WATER"
  PLC_1 (358)/2 -> Valve_2 (341)/3, Valve_1 (340)/3, Valve_3 (342)/3, Pump_3 (353)/3  "TELECONTROL"
  [POWER] -> RESIDENTIAL_1 (337)/1, Valve_1 (340)/2  "POWER"
  RESIDENTIAL_1 (337)/1 -> [RESIDENTIAL_1_QoS]  "RESIDENTIAL_QoS"
  Industrial_1 (339)/1 -> [INDUSTRIAL_1_QoS]  "RESIDENTIAL_QoS"
  Pipe_3 (345)/1 -> Industrial_1 (339)/2  "WATER"
  [RESIDENTIAL_2_QoS] -> Mux/2
  [INDUSTRIAL_1_QoS] -> Mux/3
  Tank_3 (350)/2 -> Pipe_6 (348)/1, [Water_Tank_3], Scope1/1, Pipe_3 (345)/1  "WATER"
  Tank_2 (344)/2 -> [Water_Tank_2], Pipe_2 (336)/1  "WATER"
  Constant4/1 -> Pipe_5 (347)/2  "VALVE_QoS"
  Constant13/1 -> Pipe_1 (335)/3  "PUMP_QoS"
  Dam_Water (354)/1 -> HOL_DAM (326)/2, Tank_1 (334)/2  "WATER"
  Pipe_0 (349)/1 -> Dam_Water (354)/1  "WATER"
  Max/1 -> Pipe_0 (349)/3  "PUMP_QoS"
  Constant14/1 -> Pipe_0 (349)/2  "VALVE_QoS"
  Control_Dam (329)/1 -> Pump_1 (351)/3, Pump_2 (352)/3, Dam_Plant (355)/2  "TELECONTROL"
  SCADA_Dam (356)/1 -> Min1/2, Dam_Plant (355)/1, Pump_1 (351)/1, Pump_2 (352)/1  "CYBER_FAULT"
  Pump_2 (352)/2 -> Max/1  "PUMP_QoS"
  Pump_1 (351)/2 -> Max/2  "PUMP_QoS"
  Pump_1 (351)/1 -> Min/2  "CYBER_FAULT"
  Control_Dam (329)/2 -> [CONTROL_1_QoS], HOL_DAM (326)/3  "CONTROL_QoS"
  Min1/1 -> HOL_DAM (326)/1  "CYBER_FAULT"
  SCADA_City (333)/1 -> Min4/3, Min7/1  "CYBER_FAULT"
  Tank_1 (334)/2 -> [Water_Tank_1], Pipe_4 (346)/1, Pipe_5 (347)/1, Pipe_1 (335)/1  "WATER"
  Pipe_6 (348)/1 -> Tank3_Availability (359)/1  "WATER"
  PLC_1 (358)/1 -> Min2/2, Valve_2 (341)/1, Tank_2 (344)/1, Valve_1 (340)/1, Tank_1 (334)/1, Tank_3 (350)/1, Valve_3 (342)/1, Pump_3 (353)/1  "CYBER_FAULT"
  Pump_3 (353)/2 -> Pipe_5 (347)/3  "PUMP_QoS"
  Valve_3 (342)/2 -> Pipe_3 (345)/2  "VALVE_QoS"
  Valve_2 (341)/2 -> Pipe_2 (336)/2  "VALVE_QoS"
  Valve_1 (340)/2 -> Pipe_1 (335)/2  "VALVE_QoS"
  SCADA_City (333)/2 -> Control_City (330)/1  "SCADA_QoS"
  SCADA_Dam (356)/2 -> Control_Dam (329)/1  "SCADA_QoS"
  Control_City (330)/2 -> [CONTROL_2_QoS], HOL_CITY (360)/3  "CONTROL_QoS"
  Pipe_5 (347)/1 -> Tank_3 (350)/2  "WATER"
  Pipe_4 (346)/1 -> Tank_2 (344)/2  "WATER"
  Min/1 -> Display/1, SCADA_Dam (356)/1  "CYBER_FAULT"
  Pump_2 (352)/1 -> Min/3  "CYBER_FAULT"
  HOL_DAM (326)/1 -> Min/1, Min4/2  "CYBER_FAULT"
  Min2/1 -> Display1/1, SCADA_City (333)/1  "CYBER_FAULT"
  HOL_CITY (360)/1 -> Min2/1, Min1/1, Min5/1  "CYBER_FAULT"
  Power_Availability (362)/2 -> HOL_ELE (361)/2  "POWER_QoS"
  [POWER] -> PLC_1 (358)/2, SCADA_City (333)/2  "POWER"
  [POWER] -> Pump_1 (351)/2, Pump_2 (352)/2, SCADA_Dam (356)/2  "POWER"
  [POWER] -> Industrial_1 (339)/1  "POWER"
  SCADA_Electric (357)/2 -> Control_Power (331)/1  "SCADA_QoS"
  Gas_Turbine_1 (365)/1 -> Min3/2  "CYBER_FAULT"
  Gas_Turbine_1 (365)/2 -> Power_Availability (362)/1  "POWER"
  Gas_Turbine_1 (365)/3 -> Cooling_Tower_1 (363)/3  "HOT_WATER"
  Control_Power (331)/1 -> Gas_Turbine_1 (365)/3, Cooling_Tower_1 (363)/2  "TELECONTROL"
  SCADA_Electric (357)/1 -> Min5/2, Gas_Turbine_1 (365)/1, Cooling_Tower_1 (363)/1  "CYBER_FAULT"
  Valve_3 (342)/1 -> Min7/4  "CYBER_FAULT"
  Tank_3 (350)/1 -> Min7/3  "CYBER_FAULT"
  Pump_3 (353)/1 -> Min7/2  "CYBER_FAULT"
  Min3/1 -> SCADA_Electric (357)/1  "CYBER_FAULT"
  Cooling_Tower_1 (363)/1 -> Min3/3  "CYBER_FAULT"
  HOL_ELE (361)/1 -> Min3/1, Min4/1  "CYBER_FAULT"
  Min5/1 -> HOL_ELE (361)/1  "CYBER_FAULT"
  Min4/1 -> HOL_CITY (360)/1  "CYBER_FAULT"
  Cooling_Tower_1 (363)/2 -> Min6/1  "WATER"
  Tank3_Availability (359)/1 -> HOL_CITY (360)/2, Min6/2  "WATER"
  Constant1/1 -> Pipe_6 (348)/2  "VALVE_QoS"
  Constant7/1 -> Pipe_6 (348)/3  "PUMP_QoS"
  Min7/1 -> PLC_1 (358)/1  "CYBER_FAULT"
  Control_Power (331)/2 -> [CONTROL_3_QoS], HOL_ELE (361)/3  "CONTROL_QoS"
  Constant8/1 -> Pipe_2 (336)/3  "PUMP_QoS"
  Constant9/1 -> Pipe_4 (346)/3  "PUMP_QoS"
  Constant10/1 -> Pipe_4 (346)/2  "VALVE_QoS"
  Valve_2 (341)/1 -> Min7/8  "CYBER_FAULT"
  Tank_2 (344)/1 -> Min7/7  "CYBER_FAULT"
  Valve_1 (340)/1 -> Min7/5  "CYBER_FAULT"
  Tank_1 (334)/1 -> Min7/6  "CYBER_FAULT"
  Constant2/1 -> Pipe_3 (345)/3  "PUMP_QoS"
  Min6/1 -> Gas_Turbine_1 (365)/2  "WATER"
  [CONTROL_2_QoS] -> Mux1/2
  [CONTROL_1_QoS] -> Mux1/1
  Mux1/1 -> media1/1(u)
  media1/1(y) -> SAVE_22 (22)/1  "CONTROL_QoS"
  [CONTROL_3_QoS] -> Mux1/3
  Constant5/1 -> SCADA_Electric (357)/2  "POWER"
  Tank_3 (350)/3 -> Min8/3  "IoT_measure"
  PLC_1 (358)/3 -> SCADA_City (333)/3, Display2/1  "PLC_QoS"
  Constant3/1 -> SCADA_Dam (356)/3  "PLC_QoS"
  Constant6/1 -> SCADA_Electric (357)/3  "PLC_QoS"
  Min8/1 -> PLC_1 (358)/3, Display3/1  "IoT_measure"
  Tank_1 (334)/3 -> Min8/1  "IoT_measure"
  Tank_2 (344)/3 -> Min8/2  "IoT_measure"
  Constant/1 -> Manual Switch/2
  Power_Availability (362)/1 -> Manual Switch/1  "POWER"
  Manual Switch/1 -> [POWER]  "POWER"
  Dam_Plant (355)/2 -> Pipe_0 (349)/1  "WATER"
  Dam_Plant (355)/1 -> Min/4  "CYBER_FAULT"
  [POWER] -> Valve_3 (342)/2, Pump_3 (353)/2  "POWER"
  [Water_Tank_1] -> Mux2/1
  [Water_Tank_2] -> Mux2/2
  media2/1(y) -> SAVE_23 (23)/1  "WATER"
  Mux2/1 -> media2/1(u)
  [Water_Tank_3] -> Mux2/3
